simulink model "pedulum_model_template_2021a"  (Simulink 10.3)
settings: Solver=ode4  StartTime=0.0  StopTime=10  FixedStep=0.01  RelTol=1e-3  EnableMultiTasking=on
values from neighbouring files (symbols this model uses):
  b = app.mu_data.Value    [pedulum_gui.m]
  controller_switch = app.get_value_index(app.controller_choose)    [pedulum_gui.m]
  desire_state = [app.LQR_theta.Value ... (first row only)    [pedulum_gui.m]
  discrete_switch = 2    [pedulum_gui.m]
  disturbance_amp = app.disturbance_amp_data.Value    [pedulum_gui.m]
  disturbance_rate = app.disturbance_rate_data.Value    [pedulum_gui.m]
  disturbance_switch = app.get_value_index(app.signal_choose)    [pedulum_gui.m]
  g = 9.8    [pedulum_gui.m]
  I = app.J_data.Value    [pedulum_gui.m]
  init_angle = app.init_angle_data.Value    [pedulum_gui.m]
  init_observer_state = [app.state_observer_theta.Value,                  app.state_observer_dtheta.Value,                  app.state_observer_x.Value,                  app.state_observer_dx.Value]    [pedulum_gui.m]
  init_position = app.init_position_data.Value    [pedulum_gui.m]
  l = app.length_data.Value    [pedulum_gui.m]
  linear_switch = 1    [pedulum_gui.m]
  m = app.mass_data.Value    [pedulum_gui.m]
  M = app.car_mass_data.Value    [pedulum_gui.m]
  stepsize = app.step_data.Value    [pedulum_gui.m]
undefined symbols (not defined in the file or in its folder): A, A_observer, Ad, B, B_observer, Bd, C, D, Dd, desire_out, K_LQR, K_out, K_state, L_observer, LQR_desire_state, observer_switch, Ts
settings Model: Creator=Mr-Yu  LastModifiedBy=xpp
settings SolverCC: AutoInsertRateTranBlk=on
settings DataIOCC: LimitDataPoints=on  SaveOutput=off  SignalLogging=off  DSMLogging=off  SaveTime=off  ReturnWorkspaceOutputs=on  SignalLoggingName=sigsOut
settings OptimizationCC: InitFltsAndDblsToZero=on
settings DebuggingCC: SaveWithParameterizedLinksMsg=none  SignalResolutionControl=TryResolveAllWithWarning  MultiTaskDSMMsg=warning  MultiTaskCondExecSysMsg=none
settings HardwareCC: TargetUnknown=on
settings ModelReferenceCC: EnableRefExpFcnMdlSchedulingChecks=off
settings RTWCC: DLArmComputeVersion=20.02.1
settings GRTTargetCC: TargetFcnLib=ansi_tfl_tmw.mat

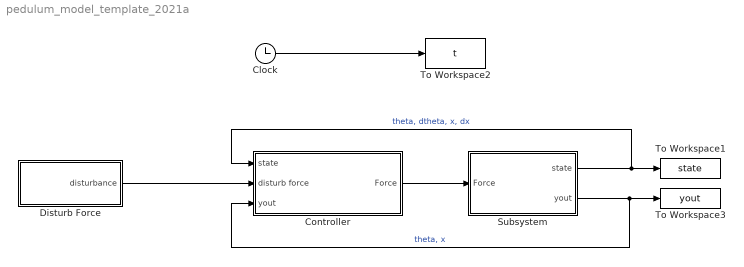
== system pedulum_model_template_2021a ==
  Clock : Clock
  Controller : Subsystem
  Disturb Force : Subsystem
  Subsystem : Subsystem
  To Workspace1 : ToWorkspace  VariableName=state  SampleTime=-1
      settings: Save2DSignal=2-D array (concatenate along first dimension)
  To Workspace2 : ToWorkspace  VariableName=t  SampleTime=-1
      settings: Save2DSignal=2-D array (concatenate along first dimension)
  To Workspace3 : ToWorkspace  VariableName=yout  SampleTime=-1
      settings: Save2DSignal=2-D array (concatenate along first dimension)
  wires:
  Disturb Force/1(disturbance) -> Controller/2(disturb force)
  Controller/1(Force) -> Subsystem/1(Force)
  Subsystem/1(state) -> Controller/1(state), To Workspace1/1  "theta, dtheta, x, dx"
  Clock/1 -> To Workspace2/1
  Subsystem/2(yout) -> Controller/3(yout), To Workspace3/1  "theta, x"

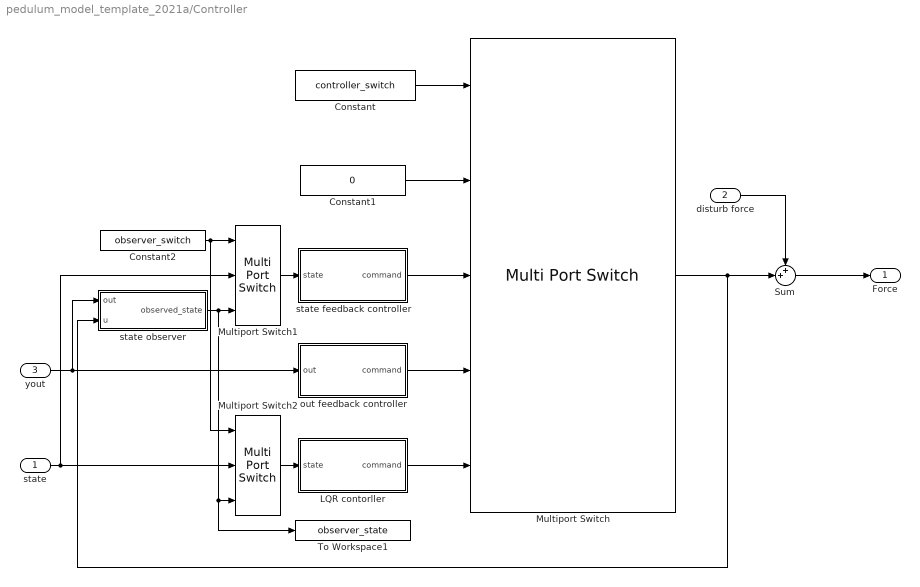
== system pedulum_model_template_2021a/Controller ==
  state : Inport
  disturb force : Inport  Port=2
  yout : Inport  Port=3
  Constant : Constant  Value=controller_switch
  Constant1 : Constant  Value=0
  Constant2 : Constant  Value=observer_switch
  LQR contorller : Subsystem
  Multiport Switch : MultiPortSwitch  Inputs=4
  Multiport Switch1 : MultiPortSwitch  DataPortOrder=Zero-based contiguous  Inputs=2  zeroidx=on
  Multiport Switch2 : MultiPortSwitch  DataPortOrder=Zero-based contiguous  Inputs=2  zeroidx=on
  Sum : Sum  Inputs=++|
  To Workspace1 : ToWorkspace  VariableName=observer_state  SampleTime=-1
      settings: Save2DSignal=2-D array (concatenate along first dimension)
  out feedback controller : Subsystem
  state feedback controller : Subsystem
  state observer : Subsystem
  Force : Outport
  wires:
  Constant/1 -> Multiport Switch/1
  state/1 -> Multiport Switch2/2, Multiport Switch1/2
  yout/1 -> out feedback controller/1(out), state observer/1(out)
  Constant1/1 -> Multiport Switch/2
  Sum/1 -> Force/1
  Multiport Switch/1 -> state observer/2(u), Sum/2
  disturb force/1 -> Sum/1
  state feedback controller/1(command) -> Multiport Switch/3
  out feedback controller/1(command) -> Multiport Switch/4
  LQR contorller/1(command) -> Multiport Switch/5
  Multiport Switch1/1 -> state feedback controller/1(state)
  state observer/1(observed_state) -> To Workspace1/1, Multiport Switch2/3, Multiport Switch1/3
  Constant2/1 -> Multiport Switch2/1, Multiport Switch1/1
  Multiport Switch2/1 -> LQR contorller/1(state)

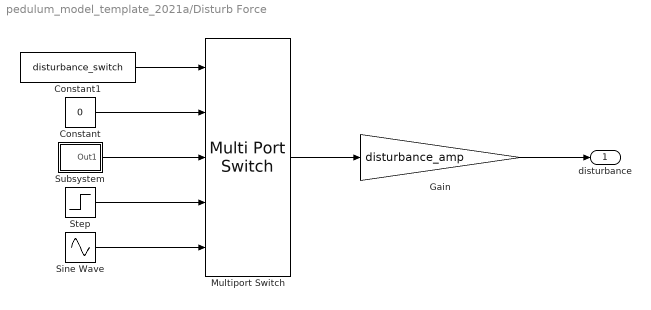
== system pedulum_model_template_2021a/Disturb Force ==
  Constant : Constant  Value=0
  Constant1 : Constant  Value=disturbance_switch
  Gain : Gain  Gain=disturbance_amp
  Multiport Switch : MultiPortSwitch  Inputs=4
  Sine Wave : Sin  Frequency=disturbance_rate  SampleTime=0
  Step : Step  Time=0  SampleTime=0
  Subsystem : Subsystem
  disturbance : Outport
  wires:
  Constant1/1 -> Multiport Switch/1
  Gain/1 -> disturbance/1
  Multiport Switch/1 -> Gain/1
  Sine Wave/1 -> Multiport Switch/5
  Constant/1 -> Multiport Switch/2
  Step/1 -> Multiport Switch/4
  Subsystem/1(Out1) -> Multiport Switch/3

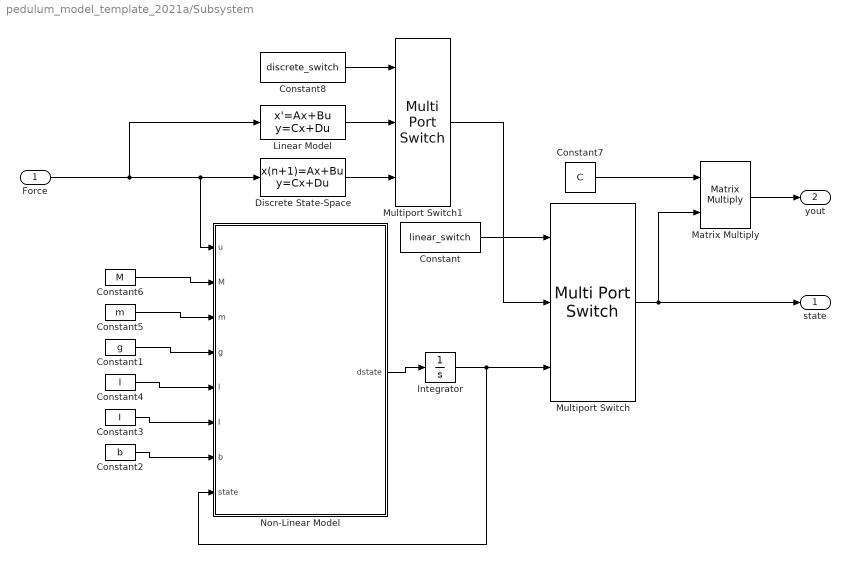
== system pedulum_model_template_2021a/Subsystem ==
  Force : Inport
  Constant : Constant  Value=linear_switch
  Constant1 : Constant  Value=g
  Constant2 : Constant  Value=b
  Constant3 : Constant  Value=I
  Constant4 : Constant  Value=l
  Constant5 : Constant  Value=m
  Constant6 : Constant  Value=M
  Constant7 : Constant  Value=C
  Constant8 : Constant  Value=discrete_switch
  Discrete State-Space : DiscreteStateSpace  A=Ad  B=Bd  C=[1, 0, 0, 0; 0, 1, 0, 0; 0, 0, 1, 0; 0, 0, 0, 1]  D=Dd  InitialCondition=[init_angle, 0, init_position, 0]  SampleTime=Ts
  Integrator : Integrator  InitialCondition=[init_angle; 0; init_position; 0]
  Linear Model : StateSpace  A=A  B=B  C=[1, 0, 0, 0; 0, 1, 0, 0; 0, 0, 1, 0; 0, 0, 0, 1]  D=D  InitialCondition=[init_angle, 0, init_position, 0]
  Matrix Multiply : Product  Multiplication=Matrix(*)
  Multiport Switch : MultiPortSwitch  Inputs=2
  Multiport Switch1 : MultiPortSwitch  Inputs=2
  Non-Linear Model : MATLAB Function  TreatAsAtomicUnit=on
  state : Outport
  yout : Outport  Port=2
  wires:
  Force/1 -> Discrete State-Space/1, Non-Linear Model/1(u), Linear Model/1
  Constant1/1 -> Non-Linear Model/4(g)
  Constant2/1 -> Non-Linear Model/7(b)
  Constant3/1 -> Non-Linear Model/6(I)
  Constant4/1 -> Non-Linear Model/5(l)
  Constant5/1 -> Non-Linear Model/3(m)
  Constant6/1 -> Non-Linear Model/2(M)
  Non-Linear Model/1(dstate) -> Integrator/1
  Multiport Switch/1 -> Matrix Multiply/2, state/1
  Constant/1 -> Multiport Switch/1
  Integrator/1 -> Multiport Switch/3, Non-Linear Model/8(state)
  Matrix Multiply/1 -> yout/1
  Constant7/1 -> Matrix Multiply/1
  Multiport Switch1/1 -> Multiport Switch/2
  Constant8/1 -> Multiport Switch1/1
  Linear Model/1 -> Multiport Switch1/2
  Discrete State-Space/1 -> Multiport Switch1/3

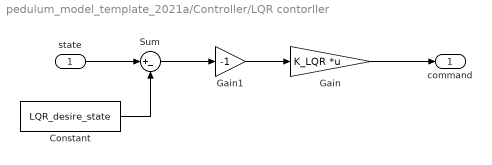
== system pedulum_model_template_2021a/Controller/LQR contorller ==
  state : Inport
  Constant : Constant  Value=LQR_desire_state
  Gain : Gain  Gain=K_LQR  Multiplication=Matrix(K*u)
  Gain1 : Gain  Gain=-1
  Sum : Sum  Inputs=|+-
  command : Outport
  wires:
  Gain1/1 -> Gain/1
  Constant/1 -> Sum/2
  Gain/1 -> command/1
  Sum/1 -> Gain1/1
  state/1 -> Sum/1

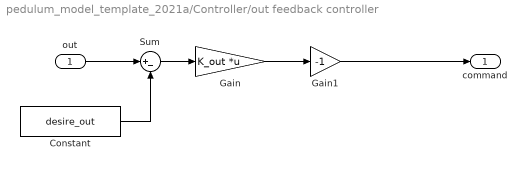
== system pedulum_model_template_2021a/Controller/out feedback controller ==
  out : Inport
  Constant : Constant  Value=desire_out
  Gain : Gain  Gain=K_out  Multiplication=Matrix(K*u)
  Gain1 : Gain  Gain=-1
  Sum : Sum  Inputs=|+-
  command : Outport
  wires:
  Gain/1 -> Gain1/1
  Gain1/1 -> command/1
  Constant/1 -> Sum/2
  Sum/1 -> Gain/1
  out/1 -> Sum/1

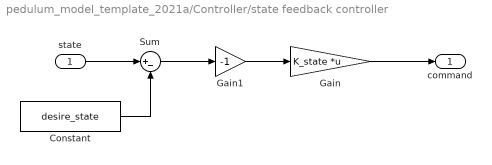
== system pedulum_model_template_2021a/Controller/state feedback controller ==
  state : Inport
  Constant : Constant  Value=desire_state
  Gain : Gain  Gain=K_state  Multiplication=Matrix(K*u)
  Gain1 : Gain  Gain=-1
  Sum : Sum  Inputs=|+-
  command : Outport
  wires:
  Constant/1 -> Sum/2
  state/1 -> Sum/1
  Sum/1 -> Gain1/1
  Gain/1 -> command/1
  Gain1/1 -> Gain/1

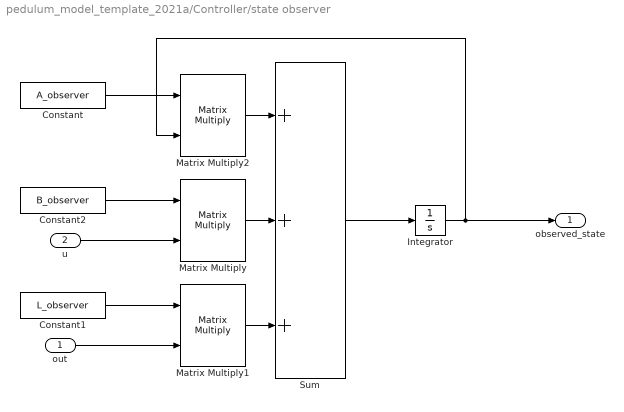
== system pedulum_model_template_2021a/Controller/state observer ==
  out : Inport
  u : Inport  Port=2
  Constant : Constant  Value=A_observer
  Constant1 : Constant  Value=L_observer
  Constant2 : Constant  Value=B_observer
  Integrator : Integrator  InitialCondition=init_observer_state(:)
  Matrix Multiply : Product  Multiplication=Matrix(*)
  Matrix Multiply1 : Product  Multiplication=Matrix(*)
  Matrix Multiply2 : Product  Multiplication=Matrix(*)
  Sum : Sum  Inputs=+++
  observed_state : Outport
  wires:
  Integrator/1 -> Matrix Multiply2/2, observed_state/1
  Sum/1 -> Integrator/1
  Matrix Multiply1/1 -> Sum/3
  Matrix Multiply/1 -> Sum/2
  Matrix Multiply2/1 -> Sum/1
  u/1 -> Matrix Multiply/2
  Constant2/1 -> Matrix Multiply/1
  Constant1/1 -> Matrix Multiply1/1
  out/1 -> Matrix Multiply1/2
  Constant/1 -> Matrix Multiply2/1

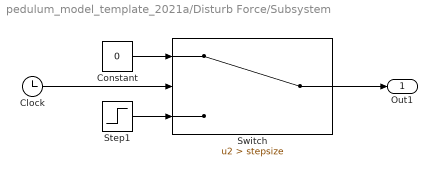
== system pedulum_model_template_2021a/Disturb Force/Subsystem ==
  Clock : Clock
  Constant : Constant  Value=0
  Step1 : Step  Time=0  After=1/stepsize  SampleTime=0
  Switch : Switch  Criteria=u2 > Threshold  Threshold=stepsize
  Out1 : Outport
  wires:
  Step1/1 -> Switch/3
  Clock/1 -> Switch/2
  Switch/1 -> Out1/1
  Constant/1 -> Switch/1

== matlab function Subsystem/Non-Linear Model ==
  data: u input double; M input double; m input double; g input double; l input double; I input double; b input double; state input double; dstate output double
function dstate = fcn(u, M, m, g, l, I, b, state)
dstate = zeros(4, 1);
theta = state(1);
dtheta = state(2);
x = state(3);
dx = state(4);
ddx = (m^2*g*l^2*sin(theta)*cos(theta) - (I + m*l^2)*(u - b*dx + m*l*sin(theta)*dtheta^2))/((m*l*cos(theta))^2 - (I + m*l^2)*(M + m));
ddtheta = -((M + m)*(m*g*l*sin(theta)) - (m*l*cos(theta))*(u - b*dx + m*l*sin(theta)*dtheta^2))/((m*l*cos(theta))^2 - (I + m*l^2)*(M + m));
dstate(1) = dtheta;
dstate(2) = ddtheta;
dstate(3) = dx;
dstate(4) = ddx;
end
